simulink model "simulink_quy_dao_v2_2020a"  (R2022b)
settings: Solver=ode8  StartTime=0.0  StopTime=400  FixedStep=0.002  RelTol=1e-3
undefined symbols (not defined in the file): K_LQR_GOC, pitch_init, roll_init, v_pitch_init, v_roll_init, v_x_init, v_y_init, v_yaw_init, v_z_init, X, x_init, Y, y_init, yaw_init, Z, z_init
libraries: sm_lib x77, nesl_utility x11, simulink x6
(part 4 of 4)

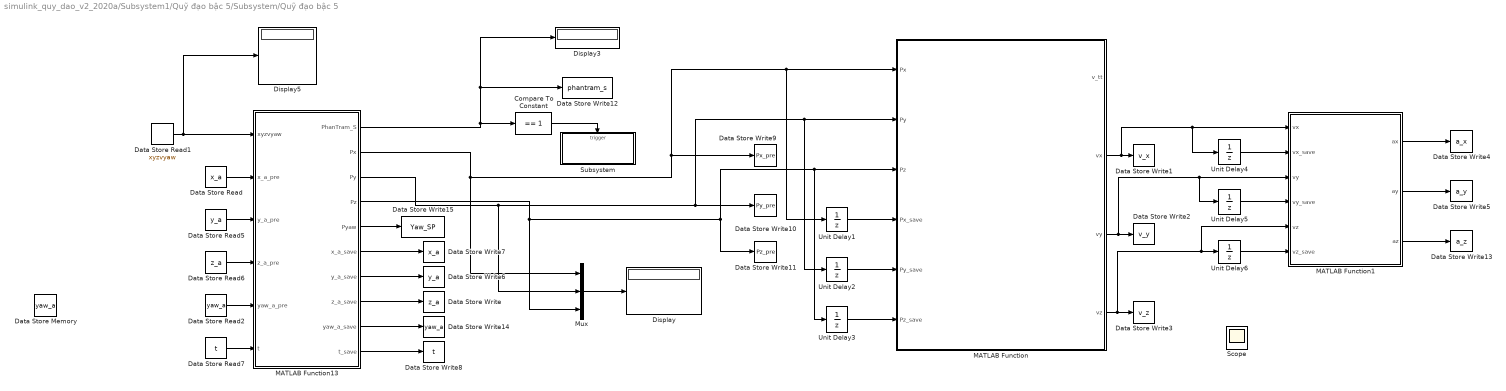
== system simulink_quy_dao_v2_2020a/Subsystem1/Quỹ đạo bậc 5/Subsystem/Quỹ đạo bậc 5 ==
  Compare To Constant : simulink/Logic and Bit Operations/Compare To Constant  relop===  const=1  OutDataTypeStr=boolean
  Data Store Memory : DataStoreMemory  DataStoreName=yaw_a  WriteAfterWriteMsg=warning  ShowAdditionalParam=off
  Data Store Read : DataStoreRead  DataStoreName=x_a  IndexOptions=Index vector (dialog)  Indices=1  OutputSizes=1
  Data Store Read1 : DataStoreRead  DataStoreName=xyzvyaw  IndexOptions=Index vector (dialog)  Indices=1  OutputSizes=1
  Data Store Read2 : DataStoreRead  DataStoreName=yaw_a  IndexOptions=Index vector (dialog)  Indices=1  OutputSizes=1
  Data Store Read5 : DataStoreRead  DataStoreName=y_a  IndexOptions=Index vector (dialog)  Indices=1  OutputSizes=1
  Data Store Read6 : DataStoreRead  DataStoreName=z_a  IndexOptions=Index vector (dialog)  Indices=1  OutputSizes=1
  Data Store Read7 : DataStoreRead  DataStoreName=t  IndexOptions=Index vector (dialog)  Indices=1  OutputSizes=1
  Data Store Write : DataStoreWrite  DataStoreName=z_a  IndexOptions=Index vector (dialog)  Indices=1  OutputSizes=1
  Data Store Write1 : DataStoreWrite  DataStoreName=v_x  IndexOptions=Index vector (dialog)  Indices=1  OutputSizes=1
  Data Store Write10 : DataStoreWrite  DataStoreName=Py_pre  IndexOptions=Index vector (dialog)  Indices=1  OutputSizes=1
  Data Store Write11 : DataStoreWrite  DataStoreName=Pz_pre  IndexOptions=Index vector (dialog)  Indices=1  OutputSizes=1
  Data Store Write12 : DataStoreWrite  DataStoreName=phantram_s  DataStoreElements=phantram_s  IndexOptions=Index vector (dialog)  Indices=1  OutputSizes=1
  Data Store Write13 : DataStoreWrite  DataStoreName=a_z  IndexOptions=Index vector (dialog)  Indices=1  OutputSizes=1
  Data Store Write14 : DataStoreWrite  DataStoreName=yaw_a  IndexOptions=Index vector (dialog)  Indices=1  OutputSizes=1
  Data Store Write15 : DataStoreWrite  DataStoreName=Yaw_SP  IndexOptions=Index vector (dialog)  Indices=1  OutputSizes=1
  Data Store Write2 : DataStoreWrite  DataStoreName=v_y  IndexOptions=Index vector (dialog)  Indices=1  OutputSizes=1
  Data Store Write3 : DataStoreWrite  DataStoreName=v_z  IndexOptions=Index vector (dialog)  Indices=1  OutputSizes=1
  Data Store Write4 : DataStoreWrite  DataStoreName=a_x  IndexOptions=Index vector (dialog)  Indices=1  OutputSizes=1
  Data Store Write5 : DataStoreWrite  DataStoreName=a_y  IndexOptions=Index vector (dialog)  Indices=1  OutputSizes=1
  Data Store Write6 : DataStoreWrite  DataStoreName=y_a  IndexOptions=Index vector (dialog)  Indices=1  OutputSizes=1
  Data Store Write7 : DataStoreWrite  DataStoreName=x_a  IndexOptions=Index vector (dialog)  Indices=1  OutputSizes=1
  Data Store Write8 : DataStoreWrite  DataStoreName=t  IndexOptions=Index vector (dialog)  Indices=1  OutputSizes=1
  Data Store Write9 : DataStoreWrite  DataStoreName=Px_pre  IndexOptions=Index vector (dialog)  Indices=1  OutputSizes=1
  Display : Display
  Display3 : Display
  Display5 : Display
  MATLAB Function : MATLAB Function  TreatAsAtomicUnit=on
  MATLAB Function1 : MATLAB Function  TreatAsAtomicUnit=on
  MATLAB Function13 : MATLAB Function  TreatAsAtomicUnit=on
  Mux : Mux  Inputs=3
  Scope : Scope
  Subsystem : Subsystem
  Unit Delay{1..6} (6 alike) : UnitDelay  SampleTime=-1  HasFrameUpgradeWarning=on
  wires:
  Compare To Constant/1 -> Subsystem/Trigger
  MATLAB Function13/1(PhanTram_S) -> Data Store Write12/1, Display3/1, Compare To Constant/1
  Data Store Read/1 -> MATLAB Function13/2(x_a_pre)
  Data Store Read6/1 -> MATLAB Function13/4(z_a_pre)
  MATLAB Function13/8(z_a_save) -> Data Store Write/1
  Data Store Read1/1 -> Display5/1, MATLAB Function13/1(xyzvyaw)
  MATLAB Function13/6(x_a_save) -> Data Store Write7/1
  MATLAB Function13/7(y_a_save) -> Data Store Write6/1
  Data Store Read5/1 -> MATLAB Function13/3(y_a_pre)
  Unit Delay4/1 -> MATLAB Function1/2(vx_save)
  MATLAB Function13/3(Py) -> Mux/2, Unit Delay2/1, MATLAB Function/2(Py), Data Store Write10/1
  Unit Delay2/1 -> MATLAB Function/5(Py_save)
  Unit Delay1/1 -> MATLAB Function/4(Px_save)
  Unit Delay3/1 -> MATLAB Function/6(Pz_save)
  Mux/1 -> Display/1
  MATLAB Function/4(vz) -> Unit Delay6/1, MATLAB Function1/5(vz), Data Store Write3/1
  MATLAB Function/3(vy) -> Unit Delay5/1, MATLAB Function1/3(vy), Data Store Write2/1
  MATLAB Function/2(vx) -> Unit Delay4/1, MATLAB Function1/1(vx), Data Store Write1/1
  MATLAB Function1/1(ax) -> Data Store Write4/1
  MATLAB Function1/2(ay) -> Data Store Write5/1
  MATLAB Function1/3(az) -> Data Store Write13/1
  Unit Delay5/1 -> MATLAB Function1/4(vy_save)
  Unit Delay6/1 -> MATLAB Function1/6(vz_save)
  MATLAB Function13/2(Px) -> Mux/1, MATLAB Function/1(Px), Unit Delay1/1, Data Store Write9/1
  MATLAB Function13/4(Pz) -> Mux/3, Data Store Write11/1, Unit Delay3/1, MATLAB Function/3(Pz)
  MATLAB Function13/10(t_save) -> Data Store Write8/1
  Data Store Read7/1 -> MATLAB Function13/6(t)
  Data Store Read2/1 -> MATLAB Function13/5(yaw_a_pre)
  MATLAB Function13/9(yaw_a_save) -> Data Store Write14/1
  MATLAB Function13/5(Pyaw) -> Data Store Write15/1

== system simulink_quy_dao_v2_2020a/Subsystem1/Quỹ đạo bậc 5/Subsystem/Quỹ đạo bậc 5/Subsystem ==
  Trigger : TriggerPort  VariantControl=Variant  PortDimensions=1
  Add : Sum
  Constant : Constant  OutDataTypeStr=double
  Data Store Read : DataStoreRead  DataStoreName=N_wp  DataStoreElements=N_wp  IndexOptions=Index vector (dialog)  Indices=1  OutputSizes=1
  Data Store Write : DataStoreWrite  DataStoreName=N_wp  DataStoreElements=N_wp  IndexOptions=Index vector (dialog)  Indices=1  OutputSizes=1
  Display : Display
  wires:
  Constant/1 -> Add/2
  Data Store Read/1 -> Add/1
  Add/1 -> Display/1, Data Store Write/1

== matlab function simulink_quy_dao_v2_2020a/Subsystem/MATLAB Function2 ==
  data: T1 input; D1 output; T2 input; T3 input; T4 input; D2 output; D3 output; D4 output
function [D1,D2,D3,D4]= fcn(T1,T2,T3,T4)
D1=(T1/11.5)*1000+1000;
D2=(T2/11.5)*1000+1000;
D3=(T3/11.5)*1000+1000;
D4=(T4/11.5)*1000+1000;

end

== matlab function simulink_quy_dao_v2_2020a/Subsystem9/Subsystem4/MATLAB Function1 ==
  data: Ux input; pitch_SP output; Uy input; yaw input; roll_SP input
function pitch_SP = fcn(Ux,Uy,yaw,roll_SP)

pitch_SP=((Ux*cos(yaw)) + (Uy*sin(yaw)))/cos(roll_SP);

end

== matlab function simulink_quy_dao_v2_2020a/Subsystem9/Subsystem1/Quỹ đạo trục z/MATLAB Function10 ==
  data: q0 input; X output; qf input; v_qd input; V output; A output
function [X,V,A]= fcn(q0,qf,v_qd)
persistent t  a0 a1 a2 a3 a4 a5 

ts=0.002; %% thời gian lấy mẫu 

tf   = qf/v_qd; %% thời gian hoàn thành quãng đường

%% Quy hoạch quỹ đạo đa thức bậc 5

v0=0; % vận tốc nam đầu
ao=0; % gia tốc ban đầu

vf=0;   % vận tốc điểm cuối
af=0;   % gia tốc điểm cuối

a0 = q0;
a1 = v0;
a2 = ao/2;
a3 = -(20*q0 - 20*qf + 12*v0*tf + 8*vf*tf + 3*ao*tf^2 - af*tf^2)/(2*tf^3);
a4 = (30*q0 - 30*qf + 16*v0*tf + 14*vf*tf + 3*ao*tf^2 - 2*af*tf^2)/(2*tf^4);
a5 = -(12*q0 - 12*qf + 6*v0*tf + 6*vf*tf + ao*tf^2 - af*tf^2)/(2*tf^5);
          

if isempty(t)    
    t = 0;
end
%% thời gian ban đầu
    t = t + ts;
%     t_out = t;
 %% Check điều kiện dừng
if(t>tf)
    t=tf;
end

%% công thức tổng quát quỹ đạo bậc 5 vị trí theo thời gian t
X= a0 + a1*t + a2*t^2 + a3*t^3 + a4*t^4 + a5*t^5;
%% công thức tổng quát quỹ đạo bậc 5 vị trí theo thời gian t
V= a1 + 2*a2*t + 3*a3*t^2 + 4*a4*t^3 + 5*a5*t^4;
%% công thức tổng quát quỹ đạo bậc 5 vị trí theo thời gian t
A=  2*a2 + 6*a3*t + 12*a4*t^2 + 20*a5*t^3;
if(qf==0)
  X=0;
  V=0;
  A=0;
 end
end

== matlab function simulink_quy_dao_v2_2020a/Subsystem9/Subsystem1/Quỹ đạo trục x/MATLAB Function10 ==
  data: q0 input; X output; qf input; v_qd input; V output; A output
function [X,V,A]= fcn(q0,qf,v_qd)
persistent t  a0 a1 a2 a3 a4 a5 

ts=0.002; %% thời gian lấy mẫu 

tf   = qf/v_qd; %% thời gian hoàn thành quãng đường

%% Quy hoạch quỹ đạo đa thức bậc 5

v0=0; % vận tốc nam đầu
ao=0; % gia tốc ban đầu

vf=0;   % vận tốc điểm cuối
af=0;   % gia tốc điểm cuối

a0 = q0;
a1 = v0;
a2 = ao/2;
a3 = -(20*q0 - 20*qf + 12*v0*tf + 8*vf*tf + 3*ao*tf^2 - af*tf^2)/(2*tf^3);
a4 = (30*q0 - 30*qf + 16*v0*tf + 14*vf*tf + 3*ao*tf^2 - 2*af*tf^2)/(2*tf^4);
a5 = -(12*q0 - 12*qf + 6*v0*tf + 6*vf*tf + ao*tf^2 - af*tf^2)/(2*tf^5);
          

if isempty(t)    
    t = 0;
end
%% thời gian ban đầu
    t = t + ts;
%     t_out = t;
 %% Check điều kiện dừng
if(t>tf)
    t=tf;
end

%% công thức tổng quát quỹ đạo bậc 5 vị trí theo thời gian t
X= a0 + a1*t + a2*t^2 + a3*t^3 + a4*t^4 + a5*t^5;
%% công thức tổng quát quỹ đạo bậc 5 vị trí theo thời gian t
V= a1 + 2*a2*t + 3*a3*t^2 + 4*a4*t^3 + 5*a5*t^4;
%% công thức tổng quát quỹ đạo bậc 5 vị trí theo thời gian t
A=  2*a2 + 6*a3*t + 12*a4*t^2 + 20*a5*t^3;
if(qf==0)
  X=0;
  V=0;
  A=0;
 end
end

== matlab function simulink_quy_dao_v2_2020a/Subsystem9/Subsystem1/Quỹ đạo trục y/MATLAB Function10 ==
  data: q0 input; X output; qf input; v_qd input; V output; A output
function [X,V,A]= fcn(q0,qf,v_qd)
persistent t  a0 a1 a2 a3 a4 a5 

ts=0.002; %% thời gian lấy mẫu 

tf   = qf/v_qd; %% thời gian hoàn thành quãng đường


%% Quy hoạch quỹ đạo đa thức bậc 5

v0=0; % vận tốc nam đầu
ao=0; % gia tốc ban đầu

vf=0;   % vận tốc điểm cuối
af=0;   % gia tốc điểm cuối

a0 = q0;
a1 = v0;
a2 = ao/2;
a3 = -(20*q0 - 20*qf + 12*v0*tf + 8*vf*tf + 3*ao*tf^2 - af*tf^2)/(2*tf^3);
a4 = (30*q0 - 30*qf + 16*v0*tf + 14*vf*tf + 3*ao*tf^2 - 2*af*tf^2)/(2*tf^4);
a5 = -(12*q0 - 12*qf + 6*v0*tf + 6*vf*tf + ao*tf^2 - af*tf^2)/(2*tf^5);
          

if isempty(t)    
    t = 0;
end
%% thời gian ban đầu
    t = t + ts;
%     t_out = t;
 %% Check điều kiện dừng
if(t>tf)
    t=tf;
end

%% công thức tổng quát quỹ đạo bậc 5 vị trí theo thời gian t
X= a0 + a1*t + a2*t^2 + a3*t^3 + a4*t^4 + a5*t^5;
%% công thức tổng quát quỹ đạo bậc 5 vị trí theo thời gian t
V= a1 + 2*a2*t + 3*a3*t^2 + 4*a4*t^3 + 5*a5*t^4;
%% công thức tổng quát quỹ đạo bậc 5 vị trí theo thời gian t
A=  2*a2 + 6*a3*t + 12*a4*t^2 + 20*a5*t^3;

if(qf==0)
  X=0;
  V=0;
  A=0;
 end
end

== matlab function simulink_quy_dao_v2_2020a/Subsystem1/G00(xyzv)/MATLAB Function1 ==
  data: xyzvyaw_in input; xyzv_out output; yaw_out output
function [xyzv_out,yaw_out]= fcn(xyzvyaw_in)
        
        x_out = xyzvyaw_in(1);
        y_out = xyzvyaw_in(2);
        z_out = xyzvyaw_in(3);
        v_out = xyzvyaw_in(4);
        yaw_out=xyzvyaw_in(5);

        xyzv_out  = [x_out ; y_out ; z_out ; v_out ; yaw_out ];
end

== matlab function simulink_quy_dao_v2_2020a/Subsystem9/Subsystem/MATLAB Function7 ==
  settings: updateMethod=DISCRETE
  data: roll input; pitch input; z_2dot_SP input; z_dot_SP input; z_SP input; a0 input; a1 input; K input; z input; z_dot input; U1 output; ez output; ez_dot output
function [U1,ez,ez_dot]= fcn(roll,pitch,z_2dot_SP,z_dot_SP,z_SP,a0,a1,K,z,z_dot)  
    %% khai báo biến hệ thống
    g=9.81;
    m=1.7;
    %% phương trình trạng thái
    % z_2dot=((U1*cos(pitch)*cos(roll))/m) - g;
    %% Chọn phương trình mặt trượt có dạng
    ez=z_SP-z;
    ez_dot=z_dot_SP-z_dot;
    Sz= a1*(z_dot_SP-z_dot)+a0*(z_SP-z);
    %% Chọn tiêu chí tốc độ hội tụ, trong đó K là hệ số dương Nếu K càng lớn thì độ hội tụ về 0 càng giảm
    VSz_dot=-K*sign(Sz);
    %% Thiết kế tín hiệu điều khiển Ux Uy
    U1=(m/(cos(roll)*cos(pitch)))*(z_2dot_SP+K*sign(Sz)*abs(Sz)+g+a0*(z_dot_SP-z_dot));
end

== matlab function simulink_quy_dao_v2_2020a/Subsystem9/Subsystem5/MATLAB Function7 ==
  data: U1 input; y_2dot_SP input; y_dot_SP input; y_SP input; a0 input; Uy output; K input; y input; y_dot input; ey output; ey_dot output
function [Uy,ey,ey_dot]= fcn(U1,y_2dot_SP,y_dot_SP,y_SP,a0,K,y,y_dot) 

%% khai báo biến hệ thống
m=1.7;

%% phương trình trạng thái

% y_2dot=-(U1*cos(yaw)*sin(roll) - cos(roll)*sin(pitch)*sin(yaw))/m;

%% Chọn phương trình mặt trượt có dạng
ey=y_SP-y;
ey_dot=y_dot_SP-y_dot;
Sy=(ey_dot)+a0*(ey);

%% Chọn tiêu chí tốc độ hội tụ, trong đó K là hệ số dương Nếu K càng lớn thì độ hội tụ về 0 càng giảm

VSy=-K*sign(Sy);

%% Thiết kế tín hiệu điều khiển Ux Uy

Uy=(m/U1)*(y_2dot_SP+a0*(y_dot_SP-y_dot)+K*sign(Sy)*abs(Sy));

end

== matlab function simulink_quy_dao_v2_2020a/Subsystem9/Subsystem5/MATLAB Function9 ==
  data: U1 input; x_2dot_SP input; x_dot_SP input; x_SP input; a0 input; K input; Ux output; x input; x_dot input; ex_dot output; ex output
function [Ux,ex_dot,ex]= fcn(U1,x_2dot_SP,x_dot_SP,x_SP,a0,K,x,x_dot) 

%% khai báo biến hệ thống

m=1.7;

%% phương trình trạng thái

% x_2dot=(U1*sin(roll)*sin(yaw) + cos(roll)*cos(yaw)*sin(pitch))/m;

%% Chọn phương trình mặt trượt có dạng
ex=x_SP-x;
ex_dot=x_dot_SP-x_dot;
Sx=(ex_dot)+a0*(ex);

%% Chọn tiêu chí tốc độ hội tụ, trong đó K là hệ số dương Nếu K càng lớn thì độ hội tụ về 0 càng giảm

VSx=-K*sign(Sx);

%% Thiết kế tín hiệu điều khiển Ux Uy

Ux=(m/U1)*(x_2dot_SP+a0*(x_dot_SP-x_dot)+K*sign(Sx)*abs(Sx));

end

== matlab function simulink_quy_dao_v2_2020a/Subsystem9/Subsystem4/MATLAB Function8 ==
  data: Ux input; roll_SP output; Uy input; yaw input
function roll_SP = fcn(Ux,Uy,yaw)

roll_SP=(Ux*sin(yaw)) - (Uy*cos(yaw));

end

== matlab function simulink_quy_dao_v2_2020a/Subsystem1/Quỹ đạo bậc 5/Subsystem/Quỹ đạo bậc 5/MATLAB Function13 ==
  data: xyzvyaw input; PhanTram_S output; Px output; Py output; Pz output; Pyaw output; x_a_save output; y_a_save output; z_a_save output; yaw_a_save output; t_save output; x_a_pre input; y_a_pre input; z_a_pre input; yaw_a_pre input; t input
function [PhanTram_S,Px,Py,Pz,Pyaw,x_a_save,y_a_save,z_a_save,yaw_a_save,t_save]= fcn(xyzvyaw,x_a_pre,y_a_pre,z_a_pre,yaw_a_pre,t)
    x_b=xyzvyaw(1);
    y_b=xyzvyaw(2);
    z_b=xyzvyaw(3);
    v_tb=xyzvyaw(4);
    yaw_b=xyzvyaw(5);
    AB = sqrt((x_b-x_a_pre)^2+(y_b-y_a_pre)^2+(z_b-z_a_pre)^2);
    if(v_tb>0)
        tf = AB/v_tb;
    else
        tf=0;
    end
    ts = 0.0015; 
    %% Nội suy Phần tram quãng đường liên tục theo thời gian theo phương pháp quy hoạch quỹ đạo bậc 3
   qf=AB;

    a_0 = 0;
    a_1 = 0;
    a_2 = 0;
    a_3 = ((20*qf)/(2*tf*tf*tf));
    a_4 = ((-30*qf)/(2*tf*tf*tf*tf));
    a_5 = ((12*qf)/(2*tf*tf*tf*tf*tf));
    if(t<tf)
        t_save=t+ts;
        temp=0;
    elseif(t>=tf)
        t_save=0;
        temp=1;
     else
        t_save=t;
        temp=0;
     end
    if(AB<=0)&&(temp==1)
        PhanTram_S = 1;
    else
        PhanTram_S=((a_0+ (a_1*t) + (a_2*t*t) + (a_3*t*t*t) + (a_4*t*t*t*t) + (a_5*t*t*t*t*t))/AB);
    end
     %%%

    %% Nội suy tọa độ theo công thức hình học.
    if(temp==1)
        Px=x_b;
        Py=y_b;
        Pz=z_b;
        Pyaw=yaw_b;

        x_a_save=x_b;
        y_a_save=y_b;
        z_a_save=z_b;
        yaw_a_save=yaw_b;
    else
        x_a_save=x_a_pre;
        y_a_save=y_a_pre;
        z_a_save=z_a_pre;
        yaw_a_save=yaw_a_pre;

        Px = x_a_pre + (x_b-x_a_pre)*PhanTram_S;
        Py = y_a_pre + (y_b-y_a_pre)*PhanTram_S;
        Pz = z_a_pre + (z_b-z_a_pre)*PhanTram_S;
        Pyaw = yaw_a_pre + (yaw_b-yaw_a_pre)*PhanTram_S;
    end

    % vx=(Px-Px_save)/ts;
    % vy=(Py-Py_save)/ts;
    % vz=(Pz-Pz_save)/ts;
    % v_tt=sqrt(vx*vx+vy*vy+vz*vz);
    % a_tt=(v_tt - v_tt_save)/ts;
    % Px_save=Px;
    % Py_save=Py;
    % Pz_save=Pz;
    % v_tt_save=v_tt;
     
end

== matlab function simulink_quy_dao_v2_2020a/Subsystem1/call1 ==
  data: N_wp input
function fcn(N_wp)
v=15;
    switch(N_wp)  
        case 1
        MoveL([0;0;30;5;0]);
        case 2
        MoveL([0;-200;30;v;pi/4]);
        case 3
        MoveL([0;-200;130;10;pi/2]);
        case 4
        MoveL([0;-500;130;v;pi/2]);
        case 5
        MoveL([0;-850;55;10;pi]);
        case 6
        MoveL([-300;-850;150;10;-pi/6]);
        case 7
        MoveL([-300;-550;115;v;-pi/6]);
        case 8
        MoveL([0;-550;150;v;-pi/2]);
        case 9
        MoveL([0;-550;30;10;-pi/2]);
        case 10
        MoveL([0;-250;30;v;-pi/2]);
        case 11
        MoveL([0;-250;130;10;pi/4]);
        case 12
        MoveL([0;0;130;v;pi/4]);
        case 13
        MoveL([0;0;0;v;0]);
    end
end

== matlab function simulink_quy_dao_v2_2020a/Subsystem1/Quỹ đạo bậc 5/Subsystem/Quỹ đạo bậc 5/MATLAB Function ==
  data: Px input; v_tt output; Py input; Pz input; Px_save input; Py_save input; Pz_save input; vx output; vy output; vz output
function [v_tt ,vx,vy,vz]= fcn(Px,Py,Pz,Px_save,Py_save,Pz_save)
  ts=0.002;
  vx=(Px-Px_save)/ts;
  vy=(Py-Py_save)/ts;
  vz=(Pz-Pz_save)/ts;
  v_tt=sqrt((vx*vx)+(vy*vy)+(vz*vz));
end

== matlab function simulink_quy_dao_v2_2020a/Subsystem1/Quỹ đạo bậc 5/Subsystem/Quỹ đạo bậc 5/MATLAB Function1 ==
  data: vx input; ax output; vx_save input; vy input; vy_save input; vz input; vz_save input; ay output; az output
function [ax,ay,az]= fcn(vx,vx_save,vy,vy_save,vz,vz_save)
    ts=0.002;
    ax=(vx-vx_save)/ts;
    ay=(vy-vy_save)/ts;
    az=(vz-vz_save)/ts;
end

== matlab function simulink_quy_dao_v2_2020a/Subsystem/MATLAB Function1 ==
  data: D1 input; T1 output; D2 input; D3 input; D4 input; T2 output; T3 output; T4 output
function [T1,T2,T3,T4]= fcn(D1,D2,D3,D4)
T1=(D1-1000)/1000*11.5;
T2=(D2-1000)/1000*11.5;
T3=(D3-1000)/1000*11.5;
T4=(D4-1000)/1000*11.5;

end

== matlab function simulink_quy_dao_v2_2020a/Subsystem6/MATLAB Function ==
  data: T1 input; x2dot output; T2 input; T3 input; T4 input; roll input; pitch input; yaw input; roll_dot input; pitch_dot input; yaw_dot input; y2dot output; z2dot output; roll2dot output; pitch2dot output; yaw2dot output; HS_MSKK input; x_dot input; y_dot input; z_dot input
function [x2dot,y2dot,z2dot,roll2dot,pitch2dot,yaw2dot]= fcn(T1,T2,T3,T4,roll,pitch,yaw,roll_dot,pitch_dot,yaw_dot,HS_MSKK,x_dot,y_dot,z_dot)
    m = 1.7; %kg
    l = 0.25; %m
    % % b = 4.74E-5;
    % % d = 2.35E-7;
    g = 9.81; %ms2
    % % to = 0.05; %Nm
    Ix = 0.0030842; %kg.m2
    Iy = 0.0030842; %kg.m2
    Iz = 0.0032315; %kg.m2
    % Ir = 1E-4; %kg.m2
    U1 = T1+T2+T3+T4;
    U2 = l*(T2-T4);
    U3 = l*(T3-T1);
    U4 = T1-T2+T3-T4;

    x2dot=(U1*(sin(roll)*sin(yaw) + cos(roll)*cos(yaw)*sin(pitch)))/m;
    y2dot=-(U1*(cos(yaw)*sin(roll) - cos(roll)*sin(pitch)*sin(yaw)))/m;
    z2dot=(U1*cos(pitch)*cos(roll))/m - g;
    roll2dot=(Iy*pitch_dot*yaw_dot - Iz*pitch_dot*yaw_dot)/Ix + U2/Ix;
    pitch2dot=U3/Iy + (-Ix*roll_dot*yaw_dot + Iz*roll_dot*yaw_dot)/Iy;
    yaw2dot=U4/Iz + (Ix*pitch_dot*roll_dot - Iy*pitch_dot*roll_dot)/Iz;

% %% Gia lap ma sat theo cong thuc ma sat tuyen tinh voi he so cho truoc la
    FX_Friction     =  -  HS_MSKK * x_dot;
    FY_Friction     =  -  HS_MSKK * y_dot;
    FZ_Friction     =  -  HS_MSKK * z_dot;
    FR_Friction     =  -  HS_MSKK * roll_dot;
    FP_Friction     =  -  HS_MSKK * pitch_dot;
    FYaw_Friction   =  -  HS_MSKK * yaw_dot;
    FX_Limit        =     HS_MSKK /10;
    FY_Limit        =     HS_MSKK /10;
    FZ_Limit        =     HS_MSKK /10;
    FR_Limit        =     HS_MSKK /10;
    FP_Limit        =     HS_MSKK /10;
    FYaw_Limit      =     HS_MSKK /10;
    
    if(FX_Friction > FX_Limit)
        FX_Friction = FX_Limit;
    end
    if(FX_Friction < -FX_Limit)
        FX_Friction = -FX_Limit;
    end
    
    if(FY_Friction > FY_Limit)
        FY_Friction = FY_Limit;
    end
    if(FY_Friction < -FY_Limit)
        FY_Friction = -FY_Limit;
    end
    
    if(FZ_Friction > FZ_Limit)
        FZ_Friction = FZ_Limit;
    end
    if(FZ_Friction < -FZ_Limit)
        FZ_Friction = -FZ_Limit;
    end
    
    if(FR_Friction > FR_Limit)
        FR_Friction = FR_Limit;
    end
    if(FR_Friction < -FR_Limit)
        FR_Friction = -FR_Limit;
    end
    
    if(FP_Friction > FP_Limit)
        FP_Friction = FP_Limit;
    end
    if(FP_Friction < -FP_Limit)
        FP_Friction = -FP_Limit;
    end
    
    if(FYaw_Friction > FYaw_Limit)
        FYaw_Friction = FYaw_Limit;
    end
    if(FYaw_Friction < -FYaw_Limit)
        FYaw_Friction = -FYaw_Limit;
    end
    
    F_x2dot           = m*x2dot     - FX_Friction;
    if((m*x2dot)*(F_x2dot)<=0)
        F_x2dot     = m*x2dot;
    end
    F_y2dot           = m*y2dot     - FY_Friction;
    if((m*y2dot)*(F_y2dot)<=0)
        F_y2dot     = m*y2dot;
    end
    F_z2dot           = m*z2dot     - FZ_Friction;
    if((m*z2dot)*(F_z2dot)<=0)
        F_z2dot     = m*z2dot;
    end
    F_roll2dot        = m*roll2dot  - FR_Friction;
    if((m*roll2dot)*(F_roll2dot)<=0)
        F_roll2dot  = m*roll2dot;
    end
    F_pitch2dot       = m*pitch2dot - FP_Friction;
    if((m*pitch2dot)*(F_pitch2dot)<=0)
        F_pitch2dot = m*pitch2dot;
    end
    F_yaw2dot         = m*yaw2dot   - FYaw_Friction;
    if((m*yaw2dot)*(F_yaw2dot)<=0)
        F_yaw2dot   = m*yaw2dot;
    end

    x2dot           = F_x2dot/m;
    y2dot           = F_y2dot/m;
    z2dot           = F_z2dot/m;
    roll2dot        = F_roll2dot/m;
    pitch2dot       = F_pitch2dot/m;
    yaw2dot         = F_yaw2dot/m;
end
